simulink library "actuator_T2_lib"  (Simulink 7.2)
settings: Solver=ode45  SolverMode=SingleTasking  StartTime=0.0  StopTime=10.0  RelTol=1e-3
undefined symbols (not defined in the file or in its folder): AILL, AILR, bias, ELLIB, ELLOB, ELRIB, ELROB, FLAPLIB, FLAPLOB, FLAPRIB, FLAPROB, GEAR, LinearizeModeOn, RUDL, RUDU, SPLLIB, SPLLOB, SPLRIB, SPLROB, STAB, SurfaceDeadbandOn, THROTL, THROTR, TrimModeOn, TrimWithStab
libraries: Servo_Model_lib x17, simulink x2
settings Model: Creator=amurch  LastModifiedBy=la1032aw

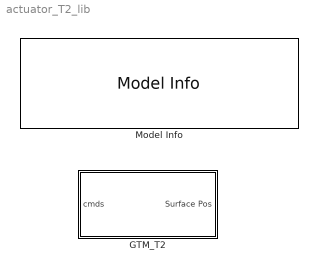
== system actuator_T2_lib ==
  GTM_T2 : Subsystem
  Model Info : simulink/Model-Wide Utilities/Model Info  SystemSampleTime=-1  InitialBlockCM=None  BlockCM=None  Frame=on  DisplayStringWithTags=|  HorizontalTextAlignment=Center  LeftAlignmentValue=0.5  SourceBlockDiagram=actuator_T2_lib  TagMaxNumber=20
      | Actuator Library
      | %<ModelVersion>
      | Las modified by %<LastModifiedBy> on %<LastModificationDate>

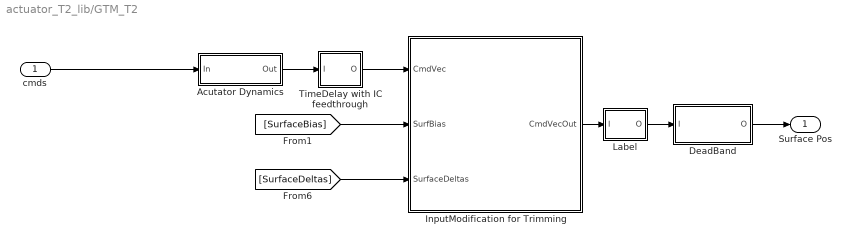
== system actuator_T2_lib/GTM_T2 ==
  cmds : Inport  OutDataType=sfix(16)  OutScaling=2^0
  Acutator Dynamics : Subsystem
  DeadBand : Subsystem
  InputModification for Trimming : Subsystem
  Label : Subsystem
  TimeDelay with IC feedthrough : Subsystem
  Surface Pos : Outport  OutDataType=sfix(16)  OutScaling=2^0
  wires:
  Acutator Dynamics/1(Out) -> TimeDelay with IC feedthrough/1(I)
  InputModification for Trimming/1(CmdVecOut) -> Label/1(I)
  [SurfaceBias] -> InputModification for Trimming/2(SurfBias)
  Label/1(O) -> DeadBand/1(I)
  [SurfaceDeltas] -> InputModification for Trimming/3(SurfaceDeltas)
  cmds/1 -> Acutator Dynamics/1(In)
  DeadBand/1(O) -> Surface Pos/1
  TimeDelay with IC feedthrough/1(O) -> InputModification for Trimming/1(CmdVec)

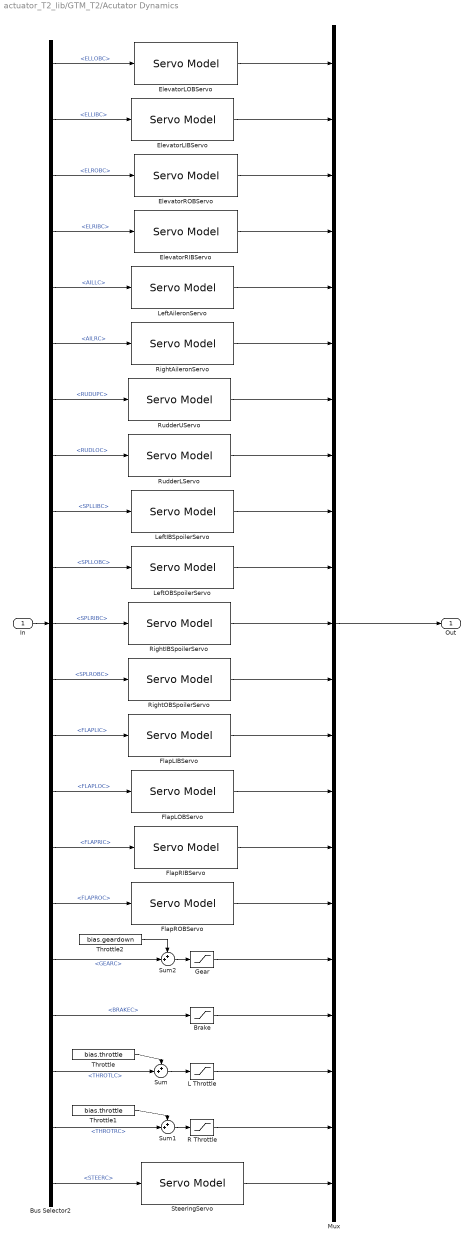
== system actuator_T2_lib/GTM_T2/Acutator Dynamics ==
  In : Inport
  Brake : Saturate  UpperLimit=1  LowerLimit=0
  Bus Selector2 : BusSelector  OutputSignals=ELLOBC,ELLIBC,ELROBC,ELRIBC,AILLC,AILRC,RUDUPC,RUDLOC,SPLLIBC,SPLLOBC,SPLRIBC,SPLROBC,FLAPLIC,FLAPLOC,FLAPRIC,FLAPROC,GEARC,BRAKEC,THROTLC,THROTRC,STEERC
  ElevatorLIBServo : Servo_Model_lib/Servo Model  SystemSampleTime=-1  freq=5  RL=300  POS_hi=20  POS_lo=-30  Bias=bias.elevator
  ElevatorLOBServo : Servo_Model_lib/Servo Model  SystemSampleTime=-1  freq=5  RL=300  POS_hi=20  POS_lo=-30  Bias=bias.elevator
  ElevatorRIBServo : Servo_Model_lib/Servo Model  SystemSampleTime=-1  freq=5  RL=300  POS_hi=20  POS_lo=-30  Bias=bias.elevator
  ElevatorROBServo : Servo_Model_lib/Servo Model  SystemSampleTime=-1  freq=5  RL=300  POS_hi=20  POS_lo=-30  Bias=bias.elevator
  FlapLIBServo : Servo_Model_lib/Servo Model  SystemSampleTime=-1  freq=5  RL=300  POS_hi=30  POS_lo=0  Bias=bias.flaps
  FlapLOBServo : Servo_Model_lib/Servo Model  SystemSampleTime=-1  freq=5  RL=300  POS_hi=30  POS_lo=0  Bias=bias.flaps
  FlapRIBServo : Servo_Model_lib/Servo Model  SystemSampleTime=-1  freq=5  RL=300  POS_hi=30  POS_lo=0  Bias=bias.flaps
  FlapROBServo : Servo_Model_lib/Servo Model  SystemSampleTime=-1  freq=5  RL=300  POS_hi=30  POS_lo=0  Bias=bias.flaps
  Gear : Saturate  UpperLimit=1  LowerLimit=0
  L Throttle : Saturate  UpperLimit=100  LowerLimit=0
  LeftAileronServo : Servo_Model_lib/Servo Model  SystemSampleTime=-1  freq=5  RL=300  POS_hi=20.0  POS_lo=-20  Bias=-1*bias.aileron
  LeftIBSpoilerServo : Servo_Model_lib/Servo Model  SystemSampleTime=-1  freq=5  RL=300  POS_hi=15  POS_lo=0  Bias=bias.speedbrake
  LeftOBSpoilerServo : Servo_Model_lib/Servo Model  SystemSampleTime=-1  freq=5  RL=300  POS_hi=45  POS_lo=0  Bias=bias.speedbrake
  Mux : Mux  Inputs=21
  R Throttle : Saturate  UpperLimit=100  LowerLimit=0
  RightAileronServo : Servo_Model_lib/Servo Model  SystemSampleTime=-1  freq=5  RL=300  POS_hi=20.0  POS_lo=-20  Bias=bias.aileron
  RightIBSpoilerServo : Servo_Model_lib/Servo Model  SystemSampleTime=-1  freq=5  RL=300  POS_hi=15  POS_lo=0  Bias=bias.speedbrake
  RightOBSpoilerServo : Servo_Model_lib/Servo Model  SystemSampleTime=-1  freq=5  RL=300  POS_hi=45  POS_lo=0  Bias=bias.speedbrake
  RudderLServo : Servo_Model_lib/Servo Model  SystemSampleTime=-1  freq=5  RL=300  POS_hi=30  POS_lo=-30.0  Bias=bias.rudder
  RudderUServo : Servo_Model_lib/Servo Model  SystemSampleTime=-1  freq=5  RL=300  POS_hi=30  POS_lo=-30.0  Bias=bias.rudder
  SteeringServo : Servo_Model_lib/Servo Model  SystemSampleTime=-1  freq=10  RL=300  POS_hi=30  POS_lo=-30  Bias=0
  Sum : Sum  Inputs=++|  OutDataType=sfix(16)  OutScaling=2^0
  Sum1 : Sum  Inputs=++|  OutDataType=sfix(16)  OutScaling=2^0
  Sum2 : Sum  Inputs=++|  OutDataType=sfix(16)  OutScaling=2^0
  Throttle : Constant  Value=bias.throttle  OutDataType=sfix(16)  OutScaling=2^0
  Throttle1 : Constant  Value=bias.throttle  OutDataType=sfix(16)  OutScaling=2^0
  Throttle2 : Constant  Value=bias.geardown  OutDataType=sfix(16)  OutScaling=2^0
  Out : Outport
  wires:
  Bus Selector2/13 -> FlapLIBServo/1  "<FLAPLIC>"
  Bus Selector2/14 -> FlapLOBServo/1  "<FLAPLOC>"
  Bus Selector2/15 -> FlapRIBServo/1  "<FLAPRIC>"
  Bus Selector2/16 -> FlapROBServo/1  "<FLAPROC>"
  Bus Selector2/18 -> Brake/1  "<BRAKEC>"
  Bus Selector2/1 -> ElevatorLOBServo/1  "<ELLOBC>"
  Bus Selector2/2 -> ElevatorLIBServo/1  "<ELLIBC>"
  ElevatorLOBServo/1 -> Mux/1
  ElevatorLIBServo/1 -> Mux/2
  Bus Selector2/3 -> ElevatorROBServo/1  "<ELROBC>"
  ElevatorROBServo/1 -> Mux/3
  Bus Selector2/4 -> ElevatorRIBServo/1  "<ELRIBC>"
  ElevatorRIBServo/1 -> Mux/4
  Bus Selector2/5 -> LeftAileronServo/1  "<AILLC>"
  LeftAileronServo/1 -> Mux/5
  Bus Selector2/6 -> RightAileronServo/1  "<AILRC>"
  RightAileronServo/1 -> Mux/6
  RudderUServo/1 -> Mux/7
  Bus Selector2/7 -> RudderUServo/1  "<RUDUPC>"
  Bus Selector2/8 -> RudderLServo/1  "<RUDLOC>"
  Bus Selector2/9 -> LeftIBSpoilerServo/1  "<SPLLIBC>"
  Bus Selector2/10 -> LeftOBSpoilerServo/1  "<SPLLOBC>"
  Bus Selector2/11 -> RightIBSpoilerServo/1  "<SPLRIBC>"
  Bus Selector2/12 -> RightOBSpoilerServo/1  "<SPLROBC>"
  RudderLServo/1 -> Mux/8
  LeftIBSpoilerServo/1 -> Mux/9
  LeftOBSpoilerServo/1 -> Mux/10
  RightIBSpoilerServo/1 -> Mux/11
  RightOBSpoilerServo/1 -> Mux/12
  FlapLIBServo/1 -> Mux/13
  FlapLOBServo/1 -> Mux/14
  FlapRIBServo/1 -> Mux/15
  FlapROBServo/1 -> Mux/16
  Bus Selector2/21 -> SteeringServo/1  "<STEERC>"
  In/1 -> Bus Selector2/1
  Mux/1 -> Out/1
  Gear/1 -> Mux/17
  Brake/1 -> Mux/18
  L Throttle/1 -> Mux/19
  R Throttle/1 -> Mux/20
  SteeringServo/1 -> Mux/21
  Sum/1 -> L Throttle/1
  Throttle/1 -> Sum/1
  Bus Selector2/19 -> Sum/2  "<THROTLC>"
  Sum1/1 -> R Throttle/1
  Throttle1/1 -> Sum1/1
  Bus Selector2/20 -> Sum1/2  "<THROTRC>"
  Sum2/1 -> Gear/1
  Throttle2/1 -> Sum2/1
  Bus Selector2/17 -> Sum2/2  "<GEARC>"

== system actuator_T2_lib/GTM_T2/DeadBand ==
  I : Inport  OutDataType=sfix(16)  OutScaling=2^0
  Deadband : Subsystem
  Flaps : Constant  Value=SurfaceDeadbandOn  OutDataType=sfix(16)  OutScaling=2^0
  Switch : Switch  Criteria=u2 ~= 0  Threshold=0.2  OutDataType=sfix(16)  OutScaling=2^0
  O : Outport  OutDataType=sfix(16)  OutScaling=2^0
  wires:
  Flaps/1 -> Switch/2
  Switch/1 -> O/1
  Deadband/1(Out) -> Switch/1
  I/1 -> Deadband/1(In), Switch/3

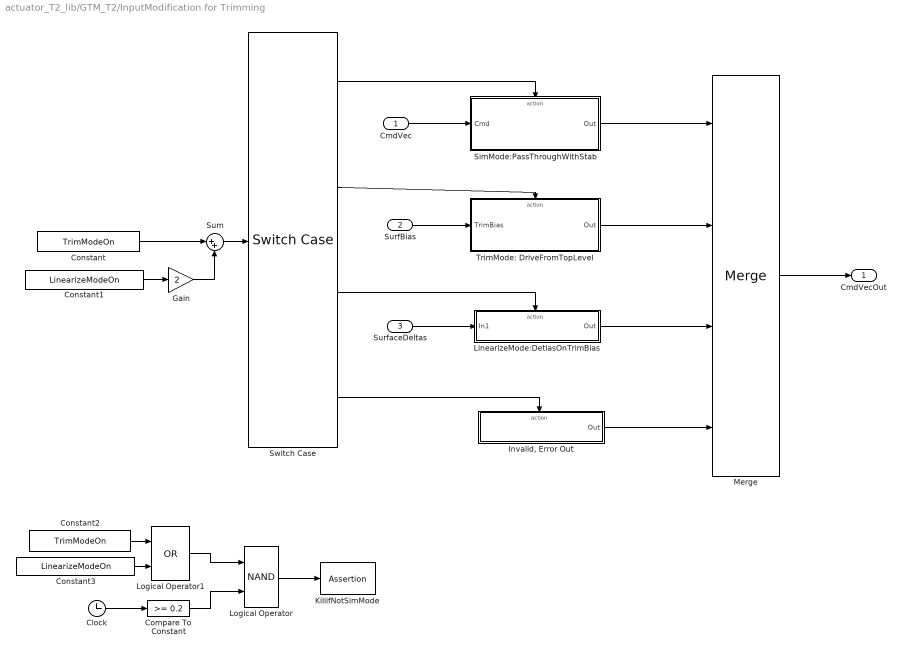
== system actuator_T2_lib/GTM_T2/InputModification for Trimming ==
  CmdVec : Inport  OutDataType=sfix(16)  OutScaling=2^0
  SurfBias : Inport  Port=2  OutDataType=sfix(16)  OutScaling=2^0
  SurfaceDeltas : Inport  Port=3  OutDataType=sfix(16)  OutScaling=2^0
  Clock : Clock
      settings: Decimation=10
  Compare To Constant : simulink/Logic and Bit Operations/Compare To Constant  SystemSampleTime=-1  relop=>=  const=0.2  LogicOutDataTypeMode=boolean  ZeroCross=off
  Constant : Constant  Value=TrimModeOn  OutDataType=sfix(16)  OutScaling=2^0
  Constant1 : Constant  Value=LinearizeModeOn  OutDataType=sfix(16)  OutScaling=2^0
  Constant2 : Constant  Value=TrimModeOn  OutDataType=sfix(16)  OutScaling=2^0
  Constant3 : Constant  Value=LinearizeModeOn  OutDataType=sfix(16)  OutScaling=2^0
  Gain : Gain  Gain=2  ParameterDataType=sfix(16)  ParameterScaling=2^0  OutDataType=sfix(16)  OutScaling=2^0
  "Invalid, Error Out" : Subsystem  TreatAsAtomicUnit=on
  KillifNotSimMode : Assertion  Enabled=on  AssertionFailFcn="warndlg('Running simulation with TrimMode or LinearizeMode engaged.  Run setup.m to reset.','Warning!')"
  LinearizeMode:DetlasOnTrimBias : Subsystem  TreatAsAtomicUnit=on
  Logical Operator : Logic  Operator=NAND  AllPortsSameDT=off  OutDataTypeMode=boolean  OutDataTypeStr=boolean
  Logical Operator1 : Logic  Operator=OR  AllPortsSameDT=off  OutDataTypeMode=boolean  OutDataTypeStr=boolean
  Merge : Merge  Inputs=4  InitialOutput=zeros(22,1)
  SimMode:PassThroughWithStab : Subsystem  TreatAsAtomicUnit=on
  Sum : Sum  Inputs=|++  OutDataType=sfix(16)  OutScaling=2^0
  Switch Case : SwitchCase  CaseConditions={0,1,2}
  TrimMode: DriveFromTopLevel : Subsystem  TreatAsAtomicUnit=on
  CmdVecOut : Outport
  wires:
  CmdVec/1 -> SimMode:PassThroughWithStab/1(Cmd)
  Switch Case/1 -> SimMode:PassThroughWithStab/Action
  Switch Case/2 -> TrimMode: DriveFromTopLevel/Action
  SurfBias/1 -> TrimMode: DriveFromTopLevel/1(TrimBias)
  SimMode:PassThroughWithStab/1(Out) -> Merge/1
  TrimMode: DriveFromTopLevel/1(Out) -> Merge/2
  Merge/1 -> CmdVecOut/1
  Switch Case/3 -> LinearizeMode:DetlasOnTrimBias/Action
  SurfaceDeltas/1 -> LinearizeMode:DetlasOnTrimBias/1(In1)
  LinearizeMode:DetlasOnTrimBias/1(Out) -> Merge/3
  Constant1/1 -> Gain/1
  Constant/1 -> Sum/1
  Gain/1 -> Sum/2
  Sum/1 -> Switch Case/1
  Switch Case/4 -> "Invalid, Error Out"/Action
  Clock/1 -> Compare To Constant/1
  Logical Operator/1 -> KillifNotSimMode/1
  Constant3/1 -> Logical Operator1/2
  Constant2/1 -> Logical Operator1/1
  Logical Operator1/1 -> Logical Operator/1
  Compare To Constant/1 -> Logical Operator/2
  "Invalid, Error Out"/1(Out) -> Merge/4

== system actuator_T2_lib/GTM_T2/Label ==
  I : Inport  OutDataType=sfix(16)  OutScaling=2^0
  Bus Creator : BusCreator  Inputs=22
  Demux : Demux  Outputs=22
  O : Outport  OutDataType=sfix(16)  OutScaling=2^0
  wires:
  I/1 -> Demux/1
  Bus Creator/1 -> O/1
  Demux/2 -> Bus Creator/2  "ELLIB"
  Demux/3 -> Bus Creator/3  "ELROB"
  Demux/4 -> Bus Creator/4  "ELRIB"
  Demux/5 -> Bus Creator/5  "AILL"
  Demux/6 -> Bus Creator/6  "AILR"
  Demux/7 -> Bus Creator/7  "RUDU"
  Demux/8 -> Bus Creator/8  "RUDL"
  Demux/9 -> Bus Creator/9  "SPLLIB"
  Demux/10 -> Bus Creator/10  "SPLLOB"
  Demux/11 -> Bus Creator/11  "SPLRIB"
  Demux/12 -> Bus Creator/12  "SPLROB"
  Demux/13 -> Bus Creator/13  "FLAPLIB"
  Demux/14 -> Bus Creator/14  "FLAPLOB"
  Demux/15 -> Bus Creator/15  "FLAPRIB"
  Demux/16 -> Bus Creator/16  "FLAPROB"
  Demux/17 -> Bus Creator/17  "STAB"
  Demux/18 -> Bus Creator/18  "GEAR"
  Demux/1 -> Bus Creator/1  "ELLOB"
  Demux/19 -> Bus Creator/19  "BRAKE"
  Demux/20 -> Bus Creator/20  "THROTL"
  Demux/21 -> Bus Creator/21  "THROTR"
  Demux/22 -> Bus Creator/22  "STEER"

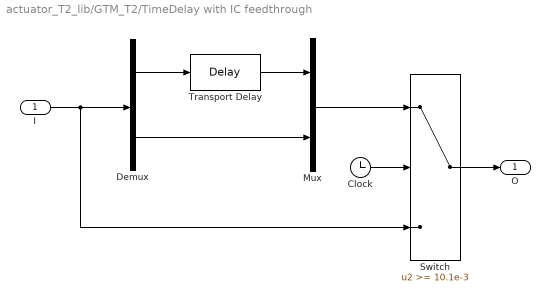
== system actuator_T2_lib/GTM_T2/TimeDelay with IC feedthrough ==
  I : Inport
  Clock : Clock
      settings: Decimation=10
  Demux : Demux  Outputs=[16 5]
  Mux : Mux  Inputs=[16 5]
  Switch : Switch  Threshold=10.1e-3  OutDataType=sfix(16)  OutScaling=2^0
  Transport Delay : TransportDelay  DelayTime=10e-3
      settings: AttributesFormatString=%<DelayTime>
  O : Outport
  wires:
  I/1 -> Switch/3, Demux/1
  Clock/1 -> Switch/2
  Switch/1 -> O/1
  Demux/1 -> Transport Delay/1
  Transport Delay/1 -> Mux/1
  Demux/2 -> Mux/2
  Mux/1 -> Switch/1

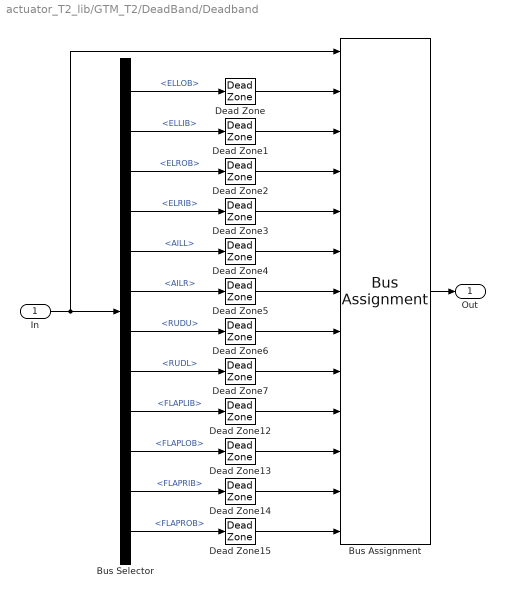
== system actuator_T2_lib/GTM_T2/DeadBand/Deadband ==
  In : Inport
  Bus Assignment : BusAssignment  AssignedSignals=ELLOB,ELLIB,ELROB,ELRIB,AILL,AILR,RUDU,RUDL,FLAPLIB,FLAPLOB,FLAPRIB,FLAPROB
  Bus Selector : BusSelector  OutputSignals=ELLOB,ELLIB,ELROB,ELRIB,AILL,AILR,RUDU,RUDL,FLAPLIB,FLAPLOB,FLAPRIB,FLAPROB
  Dead Zone : DeadZone  LowerValue=-0.3  UpperValue=0.3  SaturateOnIntegerOverflow=on
  Dead Zone1 : DeadZone  LowerValue=-0.6  UpperValue=0.6  SaturateOnIntegerOverflow=on
  Dead Zone{6,12..15} (5 alike) : DeadZone  LowerValue=-0.4  UpperValue=0.4  SaturateOnIntegerOverflow=on
  Dead Zone2 : DeadZone  LowerValue=-0.3  UpperValue=0.3  SaturateOnIntegerOverflow=on
  Dead Zone3 : DeadZone  LowerValue=-0.6  UpperValue=0.6  SaturateOnIntegerOverflow=on
  Dead Zone4 : DeadZone  LowerValue=-0.25  UpperValue=0.25  SaturateOnIntegerOverflow=on
  Dead Zone5 : DeadZone  LowerValue=-0.25  UpperValue=0.25  SaturateOnIntegerOverflow=on
  Dead Zone7 : DeadZone  LowerValue=-0.3  UpperValue=0.3  SaturateOnIntegerOverflow=on
  Out : Outport
  wires:
  Bus Assignment/1 -> Out/1
  In/1 -> Bus Selector/1, Bus Assignment/1
  Dead Zone15/1 -> Bus Assignment/13
  Dead Zone14/1 -> Bus Assignment/12
  Dead Zone13/1 -> Bus Assignment/11
  Dead Zone12/1 -> Bus Assignment/10
  Dead Zone7/1 -> Bus Assignment/9
  Dead Zone6/1 -> Bus Assignment/8
  Dead Zone5/1 -> Bus Assignment/7
  Dead Zone4/1 -> Bus Assignment/6
  Dead Zone3/1 -> Bus Assignment/5
  Dead Zone2/1 -> Bus Assignment/4
  Dead Zone1/1 -> Bus Assignment/3
  Dead Zone/1 -> Bus Assignment/2
  Bus Selector/12 -> Dead Zone15/1  "<FLAPROB>"
  Bus Selector/11 -> Dead Zone14/1  "<FLAPRIB>"
  Bus Selector/10 -> Dead Zone13/1  "<FLAPLOB>"
  Bus Selector/9 -> Dead Zone12/1  "<FLAPLIB>"
  Bus Selector/8 -> Dead Zone7/1  "<RUDL>"
  Bus Selector/7 -> Dead Zone6/1  "<RUDU>"
  Bus Selector/6 -> Dead Zone5/1  "<AILR>"
  Bus Selector/5 -> Dead Zone4/1  "<AILL>"
  Bus Selector/4 -> Dead Zone3/1  "<ELRIB>"
  Bus Selector/3 -> Dead Zone2/1  "<ELROB>"
  Bus Selector/2 -> Dead Zone1/1  "<ELLIB>"
  Bus Selector/1 -> Dead Zone/1  "<ELLOB>"

== system actuator_T2_lib/GTM_T2/InputModification for Trimming/Invalid, Error Out ==
  Action Port : ActionPort
  Constant1 : Constant  Value=zeros(22,1)  OutDataType=sfix(16)  OutScaling=2^0
  Constant2 : Constant  Value=0  OutDataType=sfix(16)  OutScaling=2^0
  InvalidMode : Assertion  Enabled=on  AssertionFailFcn="warndlg('Invalid settings for TrimMode and LinearizeMode.  Run setup.m to reset.','Warning!')"
  Out : Outport  InitialOutput=zeros(22,1)
  wires:
  Constant2/1 -> InvalidMode/1
  Constant1/1 -> Out/1

== system actuator_T2_lib/GTM_T2/InputModification for Trimming/LinearizeMode:DetlasOnTrimBias ==
  In1 : Inport  OutDataType=sfix(16)  OutScaling=2^0
  Action Port : ActionPort  ActionType=case
  Surface Allocation  For Linearizing : Subsystem
  Out : Outport  OutDataType=sfix(16)  OutScaling=2^0
  wires:
  In1/1 -> Surface Allocation  For Linearizing/1(I)
  Surface Allocation  For Linearizing/1(O) -> Out/1

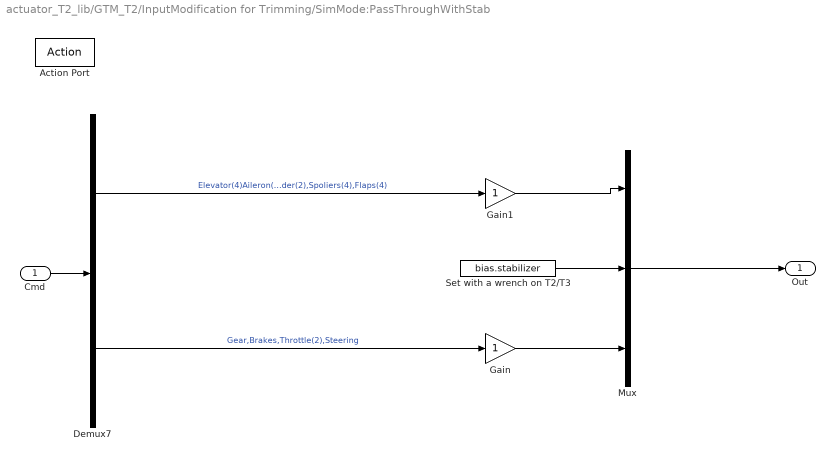
== system actuator_T2_lib/GTM_T2/InputModification for Trimming/SimMode:PassThroughWithStab ==
  Cmd : Inport  OutDataType=sfix(16)  OutScaling=2^0
  Action Port : ActionPort
  Demux7 : Demux  Outputs=[4+2+2+4+4, 1+1+2+1]
  Gain : Gain  ParameterDataType=sfix(16)  ParameterScaling=2^0  OutDataType=sfix(16)  OutScaling=2^0
  Gain1 : Gain  ParameterDataType=sfix(16)  ParameterScaling=2^0  OutDataType=sfix(16)  OutScaling=2^0
  Mux : Mux  Inputs=3
  Set with a wrench on T2/T3 : Constant  Value=bias.stabilizer  OutDataType=sfix(16)  OutScaling=2^0
  Out : Outport  OutDataType=sfix(16)  OutScaling=2^0  InitialOutput=zeros(22,1)
  wires:
  Gain/1 -> Mux/3
  Gain1/1 -> Mux/1
  Demux7/2 -> Gain/1  "Gear,Brakes,Throttle(2),Steering"
  Demux7/1 -> Gain1/1  "Elevator(4)Aileron(2),Rudder(2),Spoliers(4),Flaps(4)"
  Mux/1 -> Out/1
  Set with a wrench on T2/T3/1 -> Mux/2
  Cmd/1 -> Demux7/1

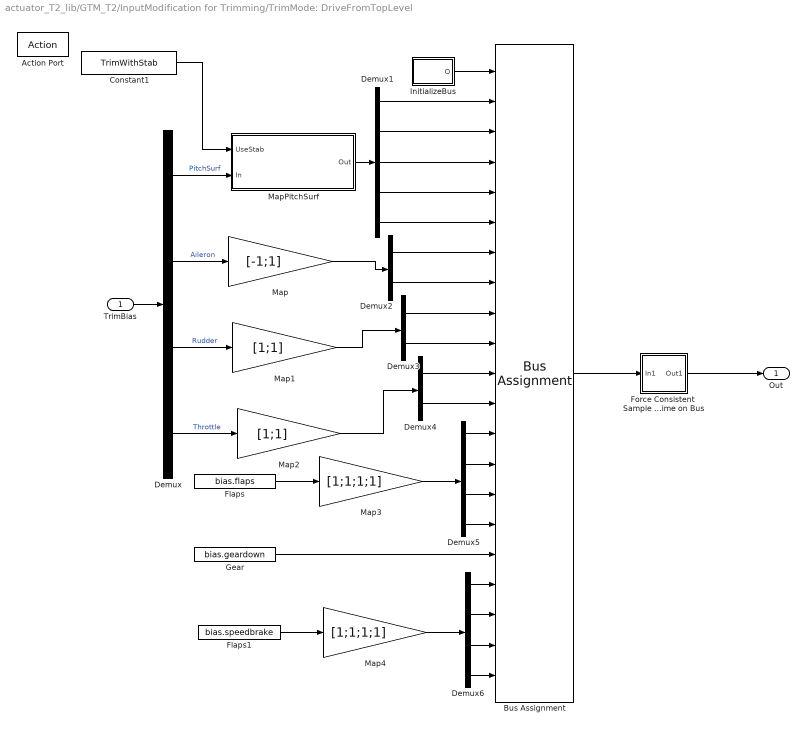
== system actuator_T2_lib/GTM_T2/InputModification for Trimming/TrimMode: DriveFromTopLevel ==
  TrimBias : Inport  OutDataType=sfix(16)  OutScaling=2^0
  Action Port : ActionPort  ActionType=case
  Bus Assignment : BusAssignment  AssignedSignals=ELLOB,ELLIB,ELROB,ELRIB,STAB,AILL,AILR,RUDU,RUDL,THROTL,THROTR,FLAPLIB,FLAPLOB,FLAPRIB,FLAPROB,GEAR,SPLLIB,SPLLOB,SPLRIB,SPLROB
  Constant1 : Constant  Value=TrimWithStab  OutDataType=sfix(16)  OutScaling=2^0
  Demux : Demux
  Demux1 : Demux  Outputs=5
  Demux2 : Demux  Outputs=2
  Demux3 : Demux  Outputs=2
  Demux4 : Demux  Outputs=2
  Demux5 : Demux
  Demux6 : Demux
  Flaps : Constant  Value=bias.flaps  OutDataType=sfix(16)  OutScaling=2^0
  Flaps1 : Constant  Value=bias.speedbrake  OutDataType=sfix(16)  OutScaling=2^0
  Force Consistent  Sample Time on Bus : Subsystem
  Gear : Constant  Value=bias.geardown  OutDataType=sfix(16)  OutScaling=2^0
  InitializeBus : Subsystem
  Map : Gain  Gain=[-1;1]  ParameterDataType=sfix(16)  ParameterScaling=2^0  OutDataType=sfix(16)  OutScaling=2^0
  Map1 : Gain  Gain=[1;1]  ParameterDataType=sfix(16)  ParameterScaling=2^0  OutDataType=sfix(16)  OutScaling=2^0
  Map2 : Gain  Gain=[1;1]  ParameterDataType=sfix(16)  ParameterScaling=2^0  OutDataType=sfix(16)  OutScaling=2^0
  Map3 : Gain  Gain=[1;1;1;1]  ParameterDataType=sfix(16)  ParameterScaling=2^0  OutDataType=sfix(16)  OutScaling=2^0
  Map4 : Gain  Gain=[1;1;1;1]  ParameterDataType=sfix(16)  ParameterScaling=2^0  OutDataType=sfix(16)  OutScaling=2^0
  MapPitchSurf : Subsystem
  Out : Outport  OutDataType=sfix(16)  OutScaling=2^0  InitialOutput=zeros(22,1)
  wires:
  TrimBias/1 -> Demux/1
  Demux/1 -> MapPitchSurf/2(In)  "PitchSurf"
  Demux/2 -> Map/1  "Aileron"
  Demux/3 -> Map1/1  "Rudder"
  Demux/4 -> Map2/1  "Throttle"
  Constant1/1 -> MapPitchSurf/1(UseStab)
  Demux1/1 -> Bus Assignment/2
  Demux1/2 -> Bus Assignment/3
  Demux1/3 -> Bus Assignment/4
  Demux1/4 -> Bus Assignment/5
  Demux1/5 -> Bus Assignment/6
  Map/1 -> Demux2/1
  Demux2/1 -> Bus Assignment/7
  Demux2/2 -> Bus Assignment/8
  Demux3/1 -> Bus Assignment/9
  Demux3/2 -> Bus Assignment/10
  Map2/1 -> Demux4/1
  Demux4/1 -> Bus Assignment/11
  Demux4/2 -> Bus Assignment/12
  Map1/1 -> Demux3/1
  Flaps/1 -> Map3/1
  Demux5/1 -> Bus Assignment/13
  Demux5/2 -> Bus Assignment/14
  Demux5/3 -> Bus Assignment/15
  Demux5/4 -> Bus Assignment/16
  Map3/1 -> Demux5/1
  Gear/1 -> Bus Assignment/17
  Flaps1/1 -> Map4/1
  Map4/1 -> Demux6/1
  Demux6/1 -> Bus Assignment/18
  Demux6/2 -> Bus Assignment/19
  Demux6/3 -> Bus Assignment/20
  Demux6/4 -> Bus Assignment/21
  MapPitchSurf/1(Out) -> Demux1/1
  InitializeBus/1(O) -> Bus Assignment/1
  Force Consistent  Sample Time on Bus/1(Out1) -> Out/1
  Bus Assignment/1 -> Force Consistent  Sample Time on Bus/1(In1)

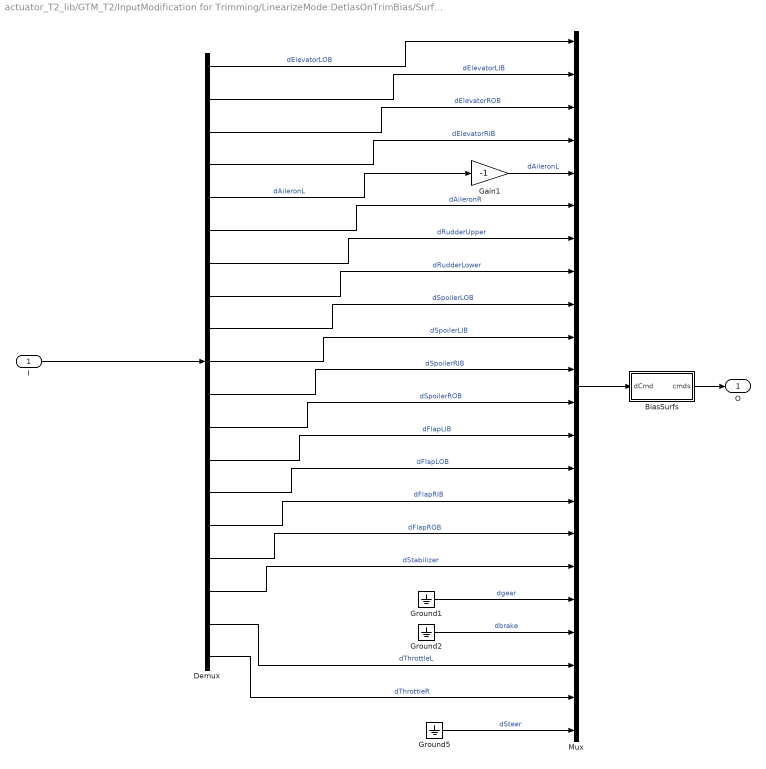
== system actuator_T2_lib/GTM_T2/InputModification for Trimming/LinearizeMode:DetlasOnTrimBias/Surface Allocation  For Linearizing ==
  I : Inport  OutDataType=sfix(16)  OutScaling=2^0
  BiasSurfs : Subsystem
  Demux : Demux  Outputs=19
  Gain1 : Gain  Gain=-1  ParameterDataType=sfix(16)  ParameterScaling=2^0  OutDataType=sfix(16)  OutScaling=2^0
  Ground1 : Ground
  Ground2 : Ground
  Ground5 : Ground
  Mux : Mux  Inputs=22
  O : Outport  OutDataType=sfix(16)  OutScaling=2^0
  wires:
  Gain1/1 -> Mux/5  "dAileronL"
  Demux/19 -> Mux/21  "dThrottleR"
  Demux/18 -> Mux/20  "dThrottleL"
  Demux/17 -> Mux/17  "dStabilizer"
  Demux/16 -> Mux/16  "dFlapROB"
  Demux/15 -> Mux/15  "dFlapRIB"
  Demux/14 -> Mux/14  "dFlapLOB"
  Demux/13 -> Mux/13  "dFlapLIB"
  Demux/12 -> Mux/12  "dSpoilerROB"
  Demux/11 -> Mux/11  "dSpoilerRIB"
  Demux/10 -> Mux/10  "dSpoilerLIB"
  Demux/9 -> Mux/9  "dSpoilerLOB"
  Demux/8 -> Mux/8  "dRudderLower"
  Demux/7 -> Mux/7  "dRudderUpper"
  Demux/6 -> Mux/6  "dAileronR"
  Demux/5 -> Gain1/1  "dAileronL"
  Demux/4 -> Mux/4  "dElevatorRIB"
  Demux/3 -> Mux/3  "dElevatorROB"
  Demux/2 -> Mux/2  "dElevatorLIB"
  Demux/1 -> Mux/1  "dElevatorLOB"
  Ground5/1 -> Mux/22  "dSteer"
  Ground2/1 -> Mux/19  "dbrake"
  Ground1/1 -> Mux/18  "dgear"
  Mux/1 -> BiasSurfs/1(dCmd)
  I/1 -> Demux/1
  BiasSurfs/1(cmds) -> O/1

== system actuator_T2_lib/GTM_T2/InputModification for Trimming/TrimMode: DriveFromTopLevel/Force Consistent  Sample Time on Bus ==
  In1 : Inport
  Bus to Vector : BusToVector
  Map4 : Gain  ParameterDataType=sfix(16)  ParameterScaling=2^0  OutDataType=sfix(16)  OutScaling=2^0
  Out1 : Outport
  wires:
  Bus to Vector/1 -> Map4/1
  Map4/1 -> Out1/1
  In1/1 -> Bus to Vector/1

== system actuator_T2_lib/GTM_T2/InputModification for Trimming/TrimMode: DriveFromTopLevel/InitializeBus ==
  Bus Creator : BusCreator  Inputs=22
  Constant : Constant  Value=zeros(22,1)  OutDataType=sfix(16)  OutScaling=2^0
  Demux : Demux  Outputs=22
  O : Outport  OutDataType=sfix(16)  OutScaling=2^0
  wires:
  Demux/1 -> Bus Creator/1  "ELLOB"
  Demux/16 -> Bus Creator/16  "FLAPROB"
  Demux/15 -> Bus Creator/15  "FLAPRIB"
  Demux/14 -> Bus Creator/14  "FLAPLOB"
  Demux/13 -> Bus Creator/13  "FLAPLIB"
  Demux/12 -> Bus Creator/12  "SPLROB"
  Demux/11 -> Bus Creator/11  "SPLRIB"
  Demux/10 -> Bus Creator/10  "SPLLOB"
  Demux/9 -> Bus Creator/9  "SPLLIB"
  Demux/8 -> Bus Creator/8  "RUDL"
  Demux/7 -> Bus Creator/7  "RUDU"
  Demux/6 -> Bus Creator/6  "AILR"
  Demux/5 -> Bus Creator/5  "AILL"
  Demux/4 -> Bus Creator/4  "ELRIB"
  Demux/3 -> Bus Creator/3  "ELROB"
  Demux/2 -> Bus Creator/2  "ELLIB"
  Bus Creator/1 -> O/1
  Demux/17 -> Bus Creator/17  "STAB"
  Demux/22 -> Bus Creator/22  "STEER"
  Demux/21 -> Bus Creator/21  "THROTR"
  Demux/20 -> Bus Creator/20  "THROTL"
  Demux/19 -> Bus Creator/19  "BRAKE"
  Demux/18 -> Bus Creator/18  "GEAR"
  Constant/1 -> Demux/1

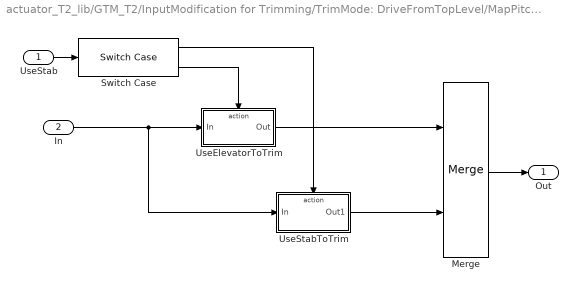
== system actuator_T2_lib/GTM_T2/InputModification for Trimming/TrimMode: DriveFromTopLevel/MapPitchSurf ==
  UseStab : Inport
  In : Inport  Port=2
  Merge : Merge
  Switch Case : SwitchCase
  UseElevatorToTrim : Subsystem  TreatAsAtomicUnit=on
  UseStabToTrim : Subsystem  TreatAsAtomicUnit=on
  Out : Outport
  wires:
  Switch Case/1 -> UseStabToTrim/Action
  UseStab/1 -> Switch Case/1
  Switch Case/2 -> UseElevatorToTrim/Action
  Merge/1 -> Out/1
  In/1 -> UseElevatorToTrim/1(In), UseStabToTrim/1(In)
  UseStabToTrim/1(Out1) -> Merge/2
  UseElevatorToTrim/1(Out) -> Merge/1

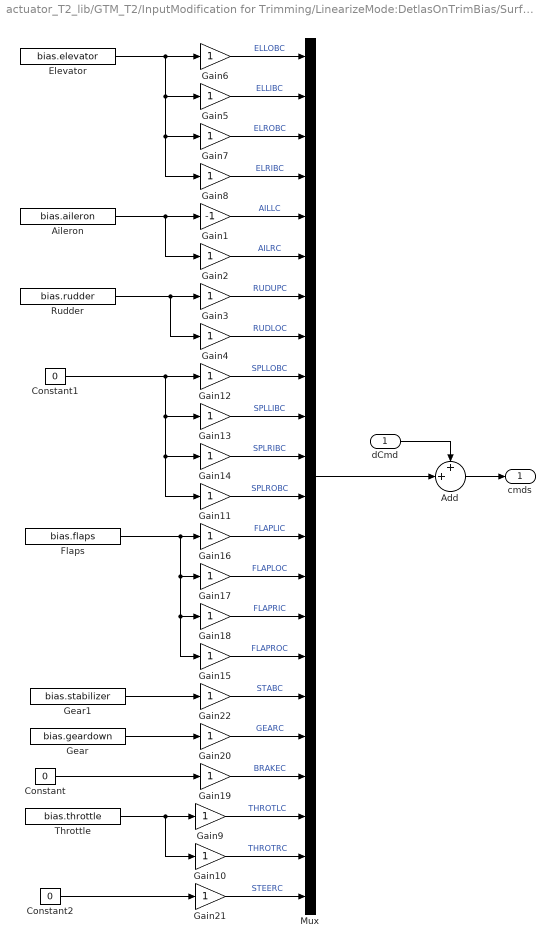
== system actuator_T2_lib/GTM_T2/InputModification for Trimming/LinearizeMode:DetlasOnTrimBias/Surface Allocation  For Linearizing/BiasSurfs ==
  dCmd : Inport  OutDataType=sfix(16)  OutScaling=2^0
  Add : Sum  Inputs=++|  OutDataType=sfix(16)  OutScaling=2^-10
  Aileron : Constant  Value=bias.aileron  OutDataType=sfix(16)  OutScaling=2^0
  Constant : Constant  Value=0  OutDataType=sfix(16)  OutScaling=2^0
  Constant1 : Constant  Value=0  OutDataType=sfix(16)  OutScaling=2^0
  Constant2 : Constant  Value=0  OutDataType=sfix(16)  OutScaling=2^0
  Elevator : Constant  Value=bias.elevator  OutDataType=sfix(16)  OutScaling=2^0
  Flaps : Constant  Value=bias.flaps  OutDataType=sfix(16)  OutScaling=2^0
  Gain1 : Gain  Gain=-1  ParameterDataType=sfix(16)  ParameterScaling=2^0  OutDataType=sfix(16)  OutScaling=2^0  SaturateOnIntegerOverflow=on  OutDataTypeStr=Inherit: Same as input  ParamDataTypeStr=Inherit: Same as input
  Gain{2..22} (21 alike) : Gain  ParameterDataType=sfix(16)  ParameterScaling=2^0  OutDataType=sfix(16)  OutScaling=2^0  SaturateOnIntegerOverflow=on  OutDataTypeStr=Inherit: Same as input  ParamDataTypeStr=Inherit: Same as input
  Gear : Constant  Value=bias.geardown  OutDataType=sfix(16)  OutScaling=2^0
  Gear1 : Constant  Value=bias.stabilizer  OutDataType=sfix(16)  OutScaling=2^0
  Mux : Mux  Inputs=22
  Rudder : Constant  Value=bias.rudder  OutDataType=sfix(16)  OutScaling=2^0
  Throttle : Constant  Value=bias.throttle  OutDataType=sfix(16)  OutScaling=2^0
  cmds : Outport  OutDataType=sfix(16)  OutScaling=2^0
  wires:
  Gain12/1 -> Mux/9  "SPLLOBC"
  Gain13/1 -> Mux/10  "SPLLIBC"
  Gain14/1 -> Mux/11  "SPLRIBC"
  Gain11/1 -> Mux/12  "SPLROBC"
  Gain16/1 -> Mux/13  "FLAPLIC"
  Gain17/1 -> Mux/14  "FLAPLOC"
  Gain18/1 -> Mux/15  "FLAPRIC"
  Gain15/1 -> Mux/16  "FLAPROC"
  Gain5/1 -> Mux/2  "ELLIBC"
  Gain6/1 -> Mux/1  "ELLOBC"
  Gain7/1 -> Mux/3  "ELROBC"
  Gain8/1 -> Mux/4  "ELRIBC"
  Gain3/1 -> Mux/7  "RUDUPC"
  Gain4/1 -> Mux/8  "RUDLOC"
  Elevator/1 -> Gain6/1, Gain5/1, Gain7/1, Gain8/1
  Rudder/1 -> Gain3/1, Gain4/1
  Flaps/1 -> Gain16/1, Gain17/1, Gain18/1, Gain15/1
  Gain19/1 -> Mux/19  "BRAKEC"
  Gear/1 -> Gain20/1
  Constant/1 -> Gain19/1
  Gain20/1 -> Mux/18  "GEARC"
  Constant1/1 -> Gain12/1, Gain13/1, Gain14/1, Gain11/1
  Gain1/1 -> Mux/5  "AILLC"
  Gain2/1 -> Mux/6  "AILRC"
  Aileron/1 -> Gain1/1, Gain2/1
  Gear1/1 -> Gain22/1
  Gain22/1 -> Mux/17  "STABC"
  Mux/1 -> Add/2
  dCmd/1 -> Add/1
  Add/1 -> cmds/1
  Gain9/1 -> Mux/20  "THROTLC"
  Gain10/1 -> Mux/21  "THROTRC"
  Throttle/1 -> Gain9/1, Gain10/1
  Constant2/1 -> Gain21/1
  Gain21/1 -> Mux/22  "STEERC"

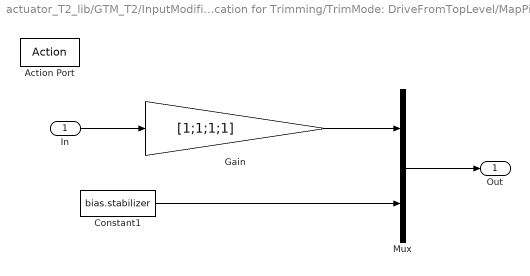
== system actuator_T2_lib/GTM_T2/InputModification for Trimming/TrimMode: DriveFromTopLevel/MapPitchSurf/UseElevatorToTrim ==
  In : Inport  OutDataType=sfix(16)  OutScaling=2^0
  Action Port : ActionPort
  Constant1 : Constant  Value=bias.stabilizer  OutDataType=sfix(16)  OutScaling=2^0
  Gain : Gain  Gain=[1;1;1;1]  ParameterDataType=sfix(16)  ParameterScaling=2^0  OutDataType=sfix(16)  OutScaling=2^0
  Mux : Mux  Inputs=[4 1]
  Out : Outport  OutDataType=sfix(16)  OutScaling=2^0  InitialOutput=[0;0;0;0;bias.stabilizer]
  wires:
  In/1 -> Gain/1
  Constant1/1 -> Mux/2
  Gain/1 -> Mux/1
  Mux/1 -> Out/1

== system actuator_T2_lib/GTM_T2/InputModification for Trimming/TrimMode: DriveFromTopLevel/MapPitchSurf/UseStabToTrim ==
  In : Inport  OutDataType=sfix(16)  OutScaling=2^0
  Action Port : ActionPort
  Constant1 : Constant  Value=bias.elevator  OutDataType=sfix(16)  OutScaling=2^0
  Gain2 : Gain  Gain=[1;1;1;1]  ParameterDataType=sfix(16)  ParameterScaling=2^0  OutDataType=sfix(16)  OutScaling=2^0
  Mux : Mux  Inputs=[4 1]
  Out1 : Outport  OutDataType=sfix(16)  OutScaling=2^0  InitialOutput=[bias.elevator*[1;1;1;1];0]
  wires:
  Constant1/1 -> Gain2/1
  In/1 -> Mux/2
  Gain2/1 -> Mux/1
  Mux/1 -> Out1/1
